simulink model "BEML_EMU"  (R2019b)
settings: configuration reference "ConfigSet_SimIntegration" (kept outside this file)
model workspace (MAT data in the model file):
  BrakesSampleTime = 0.01
  ConfigSampleTime = 0.05
  CouplingSampleTime = 0.05
  DoorsSampleTime = 0.05
  DynamicsSampleTime = 0.001
  ElectricalSampleTime = 0.05
  PRM_SimIntegration : Simulink.Parameter (value not decoded)
  PantographSampleTime = 0.05
  PneumaticsSampleTime = 0.01
  SampleTime = 0.001
  TractionSampleTime = 0.01
undefined symbols (not defined in the file): Acceleration, AngularAcceleration, AngularVelocity, BrakeFadeEnable, Brakes, BrakeShoeCoefficientCalculationMethod, BrakeShoeFrictionCoeff, BrakeTemperatureEnable, Common, DampingAdjustmentDesignMass, DavisCoeffA1, DavisCoeffA2, DavisCoeffB1, DavisCoeffB2, DavisCoefficients, DavisCoeffLeadCarC, DavisCoeffTailCarC, DiscIntNeverNeededParam, Doors, DragCalculationMethod, Dynamics, Effects, Electrical, EnableDampingAdjustmentByMass, Environment, Equipment, ExternalEffects, H, HasMotor, HasPanto, HornActivation, IsFirstVehicle, IsLastVehicle, isLeft, IsNonCab, LateralJolt, Location, LongitudinalJolt, MaxVehicles, MotionBaseSafetyCutout, OrientationDCM, P, Pantograph, Pneumatics, PneumaticsPoweredPanto, R, Traction, Transform, Tuning, UnitConfig, Velocity, VerticalJolt, VerticalJoltDown, VigilanceIntervention
libraries: simulink x35, IOStateMachinesLib x26, TestBenchLib x6, LatchesLib x3, BEML_EMU_BrakesInput_Lib x1, BEML_EMU_CBTCInterface_Lib x1, BEML_EMU_Couplers_Lib x1, BEML_EMU_DoorsInput_Lib x1, BEML_EMU_DynamicsInput_Lib x1, BEML_EMU_ElectricalInput_Lib x1, BEML_EMU_PantographInput_Lib x1, BEML_EMU_PneumaticsInput_Lib x1
(part 4 of 6)

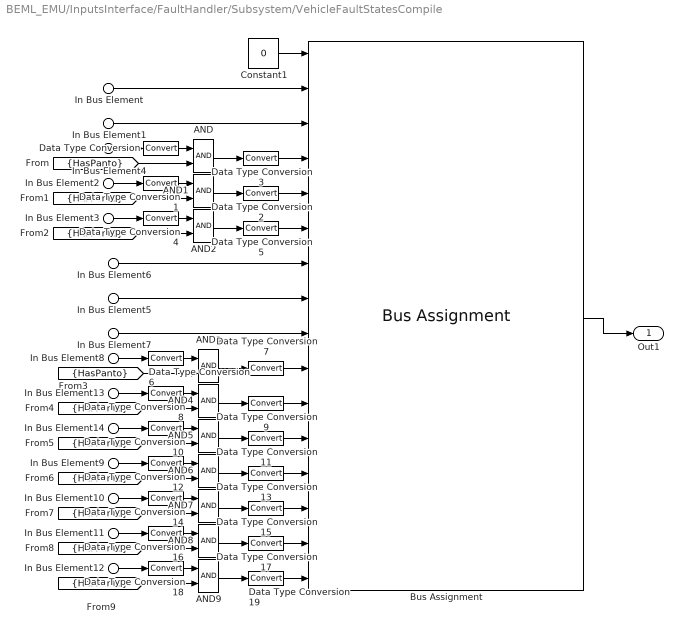
== system BEML_EMU/InputsInterface/FaultHandler/Subsystem/VehicleFaultStatesCompile ==
  In Bus Element : Inport  PortName=VehicleFaults  Element=DoorFaults.ObjectObstructingDoorWhileClosing
  In Bus Element1 : Inport  PortName=VehicleFaults  Element=DoorFaults.ObjectObstructingDoorWhileOpening
  In Bus Element4 : Inport  PortName=VehicleFaults  Element=ElectricalFaults.PantographDownForADDIntervention
  In Bus Element2 : Inport  PortName=VehicleFaults  Element=ElectricalFaults.PantographDownForORDIntervention
  In Bus Element3 : Inport  PortName=VehicleFaults  Element=ElectricalFaults.PantographRisingFailure
  In Bus Element6 : Inport  PortName=VehicleFaults  Element=ElectricalFaults.CCDetectedEmerDoorOpen
  In Bus Element7 : Inport  PortName=VehicleFaults  Element=ElectricalFaults.HVAC1EmergencyInverterTrip
  In Bus Element8 : Inport  PortName=VehicleFaults  Element=ElectricalFaults.VCBOpenedByACOvercurrent
  In Bus Element9 : Inport  PortName=VehicleFaults  Element=ElectricalFaults.VCBOpenedByMTrProtection
  In Bus Element10 : Inport  PortName=VehicleFaults  Element=ElectricalFaults.VCBOpenedByAPS
  In Bus Element11 : Inport  PortName=VehicleFaults  Element=ElectricalFaults.VCBMissingClosing
  In Bus Element12 : Inport  PortName=VehicleFaults  Element=ElectricalFaults.VCBMissingOpening
  In Bus Element13 : Inport  PortName=VehicleFaults  Element=ElectricalFaults.APSMCBGroupTripped
  In Bus Element14 : Inport  PortName=VehicleFaults  Element=ElectricalFaults.APSCircuitBreakerTripped
  In Bus Element5 : Inport  PortName=VehicleFaults  Element=TCMSFaults.MasterControllerandTrainLineIncongruence
  AND{,1..9} (10 alike) : Logic  AllPortsSameDT=off  OutDataTypeStr=boolean
  Bus Assignment : BusAssignment  AssignedSignals=DoorCloseObstruction,DoorOpenObstruction,PantographDownForADDIntervention,PantographDownForORDIntervention,PantographRaiseFailure,CCDetectDetrainmentDoorOpen,MasterControllerandTrainLineIncongruence,HVAC1EmergencyInverterTrip,VCBOpenedByACOvercurrent,MCBAPSGroupTripped,APSCircuitBreakerTripped,VCBOpenedByMTrProtection,VCBOpenedByAPS,VCBMissingClosing,VCBMissingOpening
  Constant1 : Constant  Value=0  OutDataTypeStr=Bus: BD_SimIntegration_Faults_Vehicle
  Data Type Conversion{,1..19} (20 alike) : DataTypeConversion
  Out1 : Outport
  wires:
  Constant1/1 -> Bus Assignment/1
  Bus Assignment/1 -> Out1/1
  In Bus Element/1 -> Bus Assignment/2
  In Bus Element1/1 -> Bus Assignment/3
  AND/1 -> Data Type Conversion3/1
  In Bus Element4/1 -> Data Type Conversion/1
  [HasPanto] -> AND/2
  [HasPanto] -> AND1/2
  AND1/1 -> Data Type Conversion2/1
  Data Type Conversion/1 -> AND/1
  Data Type Conversion1/1 -> AND1/1
  Data Type Conversion2/1 -> Bus Assignment/5
  Data Type Conversion3/1 -> Bus Assignment/4
  Data Type Conversion5/1 -> Bus Assignment/6
  Data Type Conversion4/1 -> AND2/1
  AND2/1 -> Data Type Conversion5/1
  In Bus Element3/1 -> Data Type Conversion4/1
  [HasPanto] -> AND2/2
  In Bus Element5/1 -> Bus Assignment/8
  In Bus Element6/1 -> Bus Assignment/7
  In Bus Element7/1 -> Bus Assignment/9
  [HasPanto] -> AND3/2
  In Bus Element8/1 -> Data Type Conversion6/1
  AND3/1 -> Data Type Conversion7/1
  Data Type Conversion6/1 -> AND3/1
  Data Type Conversion7/1 -> Bus Assignment/10
  Data Type Conversion9/1 -> Bus Assignment/11
  Data Type Conversion8/1 -> AND4/1
  AND4/1 -> Data Type Conversion9/1
  In Bus Element13/1 -> Data Type Conversion8/1
  [HasPanto] -> AND4/2
  [HasPanto] -> AND5/2
  In Bus Element14/1 -> Data Type Conversion10/1
  AND5/1 -> Data Type Conversion11/1
  Data Type Conversion10/1 -> AND5/1
  Data Type Conversion11/1 -> Bus Assignment/12
  Data Type Conversion13/1 -> Bus Assignment/13
  Data Type Conversion12/1 -> AND6/1
  AND6/1 -> Data Type Conversion13/1
  In Bus Element9/1 -> Data Type Conversion12/1
  [HasPanto] -> AND6/2
  [HasPanto] -> AND7/2
  In Bus Element10/1 -> Data Type Conversion14/1
  AND7/1 -> Data Type Conversion15/1
  Data Type Conversion14/1 -> AND7/1
  Data Type Conversion15/1 -> Bus Assignment/14
  Data Type Conversion17/1 -> Bus Assignment/15
  Data Type Conversion16/1 -> AND8/1
  AND8/1 -> Data Type Conversion17/1
  In Bus Element11/1 -> Data Type Conversion16/1
  [HasPanto] -> AND8/2
  [HasPanto] -> AND9/2
  In Bus Element12/1 -> Data Type Conversion18/1
  AND9/1 -> Data Type Conversion19/1
  Data Type Conversion18/1 -> AND9/1
  Data Type Conversion19/1 -> Bus Assignment/16
  In Bus Element2/1 -> Data Type Conversion1/1

== system BEML_EMU/InputsInterface/IOControlsInterface/InhibitsAndInternalRequests/Folding_Interlocks ==
  <RampWinder> : Inport
  RampSupport : Inport  Port=2
  GasSpring : Inport  Port=3
  <DummyCover> : Inport  Port=4
  Data Type Conversion1 : DataTypeConversion
  Data Type Conversion4 : DataTypeConversion
  NOT1 : Logic  Operator=NOT  AllPortsSameDT=off  OutDataTypeStr=boolean
  OR : Logic  Operator=OR  Inputs=3  AllPortsSameDT=off  OutDataTypeStr=boolean
  OR1 : Logic  Operator=OR  AllPortsSameDT=off  OutDataTypeStr=boolean
  InhibitDoorWinder : Outport
  InhibitRampWinder : Outport  Port=2
  wires:
  NOT1/1 -> OR1/1, OR/3
  Data Type Conversion4/1 -> InhibitDoorWinder/1
  OR/1 -> Data Type Conversion4/1
  <DummyCover>/1 -> NOT1/1
  Data Type Conversion1/1 -> InhibitRampWinder/1
  <RampWinder>/1 -> OR/2
  OR1/1 -> Data Type Conversion1/1
  RampSupport/1 -> OR1/2
  GasSpring/1 -> OR/1

== system BEML_EMU/InputsInterface/IOControlsInterface/InhibitsAndInternalRequests/Subsystem ==
  <ModeSelector> : Inport
  <ControlKey> : Inport  Port=2
  <MasterControllerHandle> : Inport  Port=3
  Compare To Constant1 : simulink/Logic and Bit Operations/Compare To Constant  relop===  const=1  OutDataTypeStr=boolean
  Compare To Constant2 : simulink/Logic and Bit Operations/Compare To Constant  relop===  const=-100  OutDataTypeStr=boolean
  Compare To Constant3 : simulink/Logic and Bit Operations/Compare To Constant  relop===  const=0  OutDataTypeStr=boolean
  Compare To Constant4 : simulink/Logic and Bit Operations/Compare To Constant  relop===  const=-100  OutDataTypeStr=boolean
  Compare To Constant5 : simulink/Logic and Bit Operations/Compare To Constant  relop===  const=0  OutDataTypeStr=boolean
  Compare To Constant6 : simulink/Logic and Bit Operations/Compare To Constant  relop===  const=5  OutDataTypeStr=boolean
  Data Type Conversion : DataTypeConversion
  Data Type Conversion1 : DataTypeConversion
  Data Type Conversion2 : DataTypeConversion
  Logical Operator1 : Logic  AllPortsSameDT=off  OutDataTypeStr=boolean
  Logical Operator2 : Logic  AllPortsSameDT=off  OutDataTypeStr=boolean
  Logical Operator3 : Logic  Operator=NOT  AllPortsSameDT=off  OutDataTypeStr=boolean
  Logical Operator4 : Logic  Operator=NOT  AllPortsSameDT=off  OutDataTypeStr=boolean
  Logical Operator5 : Logic  Operator=OR  AllPortsSameDT=off  OutDataTypeStr=boolean
  InhibitControlKey : Outport
  InhibitMS : Outport  Port=2
  InhibitMCH : Outport  Port=3
  wires:
  <ControlKey>/1 -> Compare To Constant1/1
  Compare To Constant6/1 -> Logical Operator5/2  "MS"
  Compare To Constant3/1 -> Logical Operator2/1  "MS"
  <ModeSelector>/1 -> Compare To Constant6/1, Compare To Constant5/1, Compare To Constant3/1
  Logical Operator1/1 -> Logical Operator4/1
  Logical Operator5/1 -> Data Type Conversion2/1
  Compare To Constant1/1 -> Logical Operator1/1  "Key"
  <MasterControllerHandle>/1 -> Compare To Constant4/1, Compare To Constant2/1
  Logical Operator4/1 -> Data Type Conversion1/1
  Compare To Constant2/1 -> Logical Operator1/2  "TBC"
  Logical Operator2/1 -> Logical Operator3/1
  Compare To Constant5/1 -> Logical Operator5/1  "MS"
  Logical Operator3/1 -> Data Type Conversion/1
  Compare To Constant4/1 -> Logical Operator2/2  "TBC"
  Data Type Conversion/1 -> InhibitControlKey/1
  Data Type Conversion1/1 -> InhibitMS/1
  Data Type Conversion2/1 -> InhibitMCH/1

== system BEML_EMU/InputsInterface/IOControlsInterface/InhibitsAndInternalRequests/Subsystem1 ==
  <Doors> : Inport  Partition=on  PartitionDimension=1  PartitionWidth=1  PartitionOffset=0
  Bus Selector3 : BusSelector  OutputSignals=OutputControlStates.DoorPosition
  Compare To Zero : simulink/Logic and Bit Operations/Compare To Zero  relop=>  OutDataTypeStr=boolean
  For Each : ForEach  DisableCoverage=on
  DoorsOpen : Outport  ConcatenationDimension=1
  wires:
  <Doors>/1 -> Bus Selector3/1
  Bus Selector3/1 -> Compare To Zero/1  "<DoorPosition>"
  Compare To Zero/1 -> DoorsOpen/1

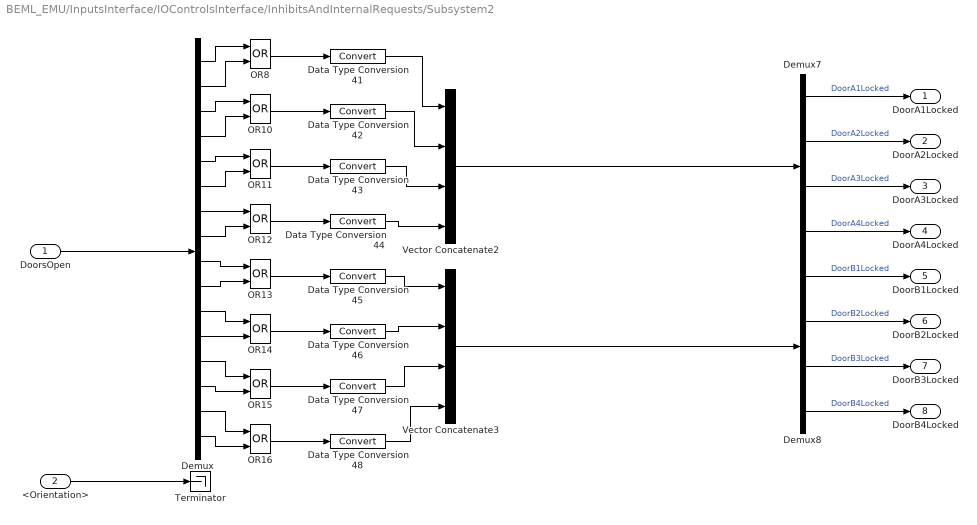
== system BEML_EMU/InputsInterface/IOControlsInterface/InhibitsAndInternalRequests/Subsystem2 ==
  DoorsOpen : Inport
  <Orientation> : Inport  Port=2
  Data Type Conversion{41..48} (8 alike) : DataTypeConversion
  Demux : Demux  Outputs=16
  Demux7 : Demux
  Demux8 : Demux
  OR{8,10..16} (8 alike) : Logic  Operator=OR  AllPortsSameDT=off  OutDataTypeStr=boolean
  Terminator : Terminator
  Vector Concatenate2 : Concatenate  NumInputs=4
  Vector Concatenate3 : Concatenate  NumInputs=4
  DoorA1Locked : Outport
  DoorA2Locked : Outport  Port=2
  DoorA3Locked : Outport  Port=3
  DoorA4Locked : Outport  Port=4
  DoorB1Locked : Outport  Port=5
  DoorB2Locked : Outport  Port=6
  DoorB3Locked : Outport  Port=7
  DoorB4Locked : Outport  Port=8
  wires:
  Demux/8 -> OR12/2
  OR13/1 -> Data Type Conversion45/1
  Data Type Conversion47/1 -> Vector Concatenate3/3
  Demux/2 -> OR8/2
  Demux/9 -> OR13/1
  Data Type Conversion48/1 -> Vector Concatenate3/4
  Demux/15 -> OR16/1
  Data Type Conversion46/1 -> Vector Concatenate3/2
  Demux/16 -> OR16/2
  Data Type Conversion45/1 -> Vector Concatenate3/1
  OR14/1 -> Data Type Conversion46/1
  Demux7/3 -> DoorA3Locked/1  "DoorA3Locked"
  Demux/4 -> OR10/2
  OR16/1 -> Data Type Conversion48/1
  Demux/10 -> OR13/2
  OR11/1 -> Data Type Conversion43/1
  Demux/11 -> OR14/1
  Demux8/1 -> DoorB1Locked/1  "DoorB1Locked"
  Demux7/4 -> DoorA4Locked/1  "DoorA4Locked"
  Demux/14 -> OR15/2
  Demux/7 -> OR12/1
  Demux/12 -> OR14/2
  Demux7/2 -> DoorA2Locked/1  "DoorA2Locked"
  Demux/6 -> OR11/2
  Demux/3 -> OR10/1
  Data Type Conversion41/1 -> Vector Concatenate2/1
  Demux/1 -> OR8/1
  Vector Concatenate2/1 -> Demux7/1
  Demux/5 -> OR11/1
  OR10/1 -> Data Type Conversion42/1
  OR8/1 -> Data Type Conversion41/1
  Demux8/4 -> DoorB4Locked/1  "DoorB4Locked"
  OR15/1 -> Data Type Conversion47/1
  Data Type Conversion42/1 -> Vector Concatenate2/2
  OR12/1 -> Data Type Conversion44/1
  Demux/13 -> OR15/1
  Vector Concatenate3/1 -> Demux8/1
  Demux8/3 -> DoorB3Locked/1  "DoorB3Locked"
  Data Type Conversion44/1 -> Vector Concatenate2/4
  Data Type Conversion43/1 -> Vector Concatenate2/3
  Demux8/2 -> DoorB2Locked/1  "DoorB2Locked"
  DoorsOpen/1 -> Demux/1
  <Orientation>/1 -> Terminator/1
  Demux7/1 -> DoorA1Locked/1  "DoorA1Locked"

== system BEML_EMU/InputsInterface/IOControlsInterface/InhibitsAndInternalRequests/Unfolding_interlocks ==
  note: when either of Winder is active, inhibit all the controls
  <RampCoverLockingLever> : Inport
  <SafetyCover> : Inport  Port=2
  <RampCover> : Inport  Port=3
  <DummyCover> : Inport  Port=4
  EDELR : Inport  Port=5
  AND : Logic  AllPortsSameDT=off  OutDataTypeStr=boolean
  Bus Selector : BusSelector  OutputSignals=Doors.EmerDoorLatched
  Data Type Conversion{,1..3} (4 alike) : DataTypeConversion
  NOT{,1..4} (5 alike) : Logic  Operator=NOT  AllPortsSameDT=off  OutDataTypeStr=boolean
  OR1 : Logic  Operator=OR  AllPortsSameDT=off  OutDataTypeStr=boolean
  InhibitSafetyCover : Outport  OutputWhenDisabled=reset  InitialOutput=1
  InhibitLockingLever : Outport  Port=2  OutputWhenDisabled=reset  InitialOutput=1
  InhibitRampCover : Outport  Port=3  OutputWhenDisabled=reset  InitialOutput=1
  InhibitRampHandle : Outport  Port=4  OutputWhenDisabled=reset  InitialOutput=1
  wires:
  <RampCover>/1 -> NOT2/1
  AND/1 -> NOT1/1
  <SafetyCover>/1 -> OR1/2, AND/1
  EDELR/1 -> Bus Selector/1
  <DummyCover>/1 -> NOT/1
  <RampCoverLockingLever>/1 -> NOT3/1
  NOT/1 -> OR1/1
  OR1/1 -> Data Type Conversion/1
  NOT2/1 -> Data Type Conversion2/1
  NOT3/1 -> Data Type Conversion3/1
  NOT1/1 -> Data Type Conversion1/1
  Data Type Conversion/1 -> InhibitSafetyCover/1
  Data Type Conversion2/1 -> InhibitRampHandle/1
  Data Type Conversion3/1 -> InhibitRampCover/1
  Data Type Conversion1/1 -> InhibitLockingLever/1
  NOT4/1 -> AND/2
  Bus Selector/1 -> NOT4/1  "<EmerDoorLatched>"

== system BEML_EMU/InputsInterface/VehicleConfigProcessing/VehicleConfigInterface/VehicleConfigInterface ==
  VehicleConfig : Inport  Partition=on  PartitionDimension=1  PartitionWidth=1  PartitionOffset=0
  VehicleUpEnabled : Inport  Port=2  Partition=on  PartitionDimension=1  PartitionWidth=1  PartitionOffset=0
  VehicleDownEnabled : Inport  Port=3  Partition=on  PartitionDimension=1  PartitionWidth=1  PartitionOffset=0
  ClassDown : Inport  Port=4  Partition=on  PartitionDimension=1  PartitionWidth=1  PartitionOffset=0
  ClassUp : Inport  Port=5  Partition=on  PartitionDimension=1  PartitionWidth=1  PartitionOffset=0
  TrainInput : Inport  Port=6
  UnitID : Inport  Port=7  Partition=on  PartitionDimension=1  PartitionWidth=1  PartitionOffset=0
  MaxUnits : Inport  Port=8
  AssignBrakes : Subsystem
  AssignDoors : Subsystem
  AssignElectrical : Subsystem
  AssignEquipment : Subsystem
  AssignPanto : Subsystem
  AssignPneumatics : Subsystem
  AssignTraction : Subsystem
  Bus Assignment1 : BusAssignment  AssignedSignals=Common,Location,Dynamics,Brakes,Pneumatics,Traction,Pantograph,Doors,Electrical,Equipment
  Bus Selector : BusSelector  OutputSignals=Dynamics
  Bus Selector1 : BusSelector  OutputSignals=Common
  Bus Selector2 : BusSelector  OutputSignals=Common.Enabled
  Bus Selector4 : BusSelector  OutputSignals=Brakes
  Common : Subsystem
  Constant1 : Constant  Value=0  OutDataTypeStr=Bus: BD_SimIntegration_Cfg_Vehicle
  Dynamics : Subsystem
  For Each : ForEach  DisableCoverage=on  ShowIterationIndex=on
  LocationConfig : Subsystem
  VehicleConfigProcessed : Outport  ConcatenationDimension=1  VectorParamsAs1DForOutWhenUnconnected=off
  Enable : Outport  Port=2  ConcatenationDimension=1
  UnitConn : Outport  Port=3  ConcatenationDimension=1
  wires:
  Bus Selector4/1 -> AssignBrakes/1(Input)  "<Brakes>"
  Bus Selector1/1 -> Common/1(Input)  "<Common>"
  TrainInput/1 -> Dynamics/2(TrainInput)
  Dynamics/1(DynamicsProcessed) -> Bus Assignment1/4  "Dynamics"
  LocationConfig/1(LocationConfig) -> Bus Assignment1/3  "Location"
  VehicleDownEnabled/1 -> LocationConfig/3(VehicleEnabledDown)
  VehicleUpEnabled/1 -> LocationConfig/2(VehicleEnabledUp)
  Bus Selector2/1 -> LocationConfig/1(VehicleEnabled)  "<Enabled>"
  Bus Selector/1 -> Dynamics/1(Dynamics)  "<Dynamics>"
  Constant1/1 -> Bus Assignment1/1
  Bus Assignment1/1 -> VehicleConfigProcessed/1  "VehicleConfig"
  VehicleConfig/1 -> AssignPneumatics/1(VehicleConfig), AssignTraction/1(VehicleConfig), AssignPanto/1(VehicleConfig), AssignDoors/1(VehicleConfig), AssignEquipment/1(VehicleConfig), AssignElectrical/1(VehicleConfig), Bus Selector4/1, Bus Selector/1, LocationConfig/7(VehicleConfig), Bus Selector2/1, Bus Selector1/1
  AssignBrakes/1(EquipmentBus) -> Bus Assignment1/5  "Brakes"
  AssignPneumatics/1(PneumaticsBus) -> Bus Assignment1/6  "Pneumatics"
  AssignTraction/1(TractionBus) -> Bus Assignment1/7  "Traction"
  AssignPanto/1(PantoBus) -> Bus Assignment1/8  "Pantograph"
  AssignElectrical/1(ElectricalBus) -> Bus Assignment1/10  "Electrical"
  AssignDoors/1(Doors) -> Bus Assignment1/9
  AssignEquipment/1(EquipmentBus) -> Bus Assignment1/11  "Equipment"
  For Each/1 -> AssignElectrical/2(Index)
  ClassDown/1 -> LocationConfig/4(ClassDown)
  ClassUp/1 -> LocationConfig/5(ClassUp)
  LocationConfig/2(Enabled) -> Enable/1
  LocationConfig/3(UnitConnection) -> UnitConn/1
  UnitID/1 -> LocationConfig/6(UnitID)
  Common/1(Common) -> Bus Assignment1/2  "Brakes"
  MaxUnits/1 -> LocationConfig/8(MaxUnit)

== system BEML_EMU/InputsInterface/VehicleConfigProcessing/VehicleConfigInterface/VehicleEnabled ==
  VehicleConfig : Inport
  Constant : Constant  Value=false  OutDataTypeStr=boolean
  Constant1 : Constant  Value=0  OutDataTypeStr=int32
  Data Type Conversion : DataTypeConversion  OutDataTypeStr=int32
  SelectDown : Selector  InputPortWidth=MaxVehicles+2  IndexOptions=Starting index (dialog)  Indices=3  OutputSizes=MaxVehicles
  SelectDown1 : Selector  InputPortWidth=MaxVehicles+2  IndexOptions=Starting index (dialog)  Indices=3  OutputSizes=MaxVehicles
  SelectUp : Selector  InputPortWidth=MaxVehicles+2  IndexOptions=Starting index (dialog)  Indices=1  OutputSizes=MaxVehicles
  SelectUp1 : Selector  InputPortWidth=MaxVehicles+2  IndexOptions=Starting index (dialog)  Indices=1  OutputSizes=MaxVehicles
  Subsystem : Subsystem
  Subsystem1 : Subsystem
  Vector Concatenate : Concatenate  NumInputs=3
  Vector Concatenate1 : Concatenate  NumInputs=3
  VehicleEnabledUp : Outport  VectorParamsAs1DForOutWhenUnconnected=off
  VehicleEnabledDown : Outport  Port=2  VectorParamsAs1DForOutWhenUnconnected=off
  VehicleClassDown : Outport  Port=3  VectorParamsAs1DForOutWhenUnconnected=off
  VehicleClassUp : Outport  Port=4  VectorParamsAs1DForOutWhenUnconnected=off
  wires:
  SelectUp/1 -> VehicleEnabledUp/1
  SelectDown/1 -> VehicleEnabledDown/1
  Subsystem/1(Enabled) -> Vector Concatenate/2
  Vector Concatenate/1 -> SelectDown/1, SelectUp/1
  Constant/1 -> Vector Concatenate/3, Vector Concatenate/1
  VehicleConfig/1 -> Subsystem1/1(VehicleConfig), Subsystem/1(VehicleConfig)
  Subsystem1/1(Class) -> Data Type Conversion/1
  Vector Concatenate1/1 -> SelectDown1/1, SelectUp1/1
  SelectDown1/1 -> VehicleClassDown/1
  Data Type Conversion/1 -> Vector Concatenate1/2
  Constant1/1 -> Vector Concatenate1/3, Vector Concatenate1/1
  SelectUp1/1 -> VehicleClassUp/1

== system BEML_EMU/SimulatorSystems/AudioSystemInterface/Subsystem1/For Each Subsystem ==
  Doors : Inport  Partition=on  PartitionDimension=1  PartitionWidth=1  PartitionOffset=0
  Bus Selector : BusSelector  OutputSignals=Audio.DoorOpening,Audio.DoorClosing,Audio.DoorOpeningAlarm,Audio.DoorClosingAlarm,Audio.DoorEmergencyReleased
  For Each : ForEach  DisableCoverage=on
  OR : Logic  Operator=OR  AllPortsSameDT=off  OutDataTypeStr=boolean
  Opening : Outport  ConcatenationDimension=1
  Closing : Outport  Port=2  ConcatenationDimension=1
  OpeningorClosingAlarm : Outport  Port=3  ConcatenationDimension=1
  EED_EADOperated : Outport  Port=4  ConcatenationDimension=1
  wires:
  Doors/1 -> Bus Selector/1
  Bus Selector/1 -> Opening/1  "<DoorOpening>"
  Bus Selector/2 -> Closing/1  "<DoorClosing>"
  OR/1 -> OpeningorClosingAlarm/1
  Bus Selector/3 -> OR/1  "<DoorOpeningAlarm>"
  Bus Selector/4 -> OR/2  "<DoorClosingAlarm>"
  Bus Selector/5 -> EED_EADOperated/1  "<DoorEmergencyReleased>"

== system BEML_EMU/SimulatorSystems/AudioSystemInterface/Subsystem1/For Each Subsystem1 ==
  Traction : Inport  Partition=on  PartitionDimension=1  PartitionWidth=1  PartitionOffset=0
  Bus Selector1 : BusSelector  OutputSignals=TCUSlipDetected,TCUSlideDetected
  For Each : ForEach  DisableCoverage=on
  Slip : Outport  ConcatenationDimension=1
  Slide : Outport  Port=2  ConcatenationDimension=1
  wires:
  Bus Selector1/2 -> Slide/1  "<TCUSlideDetected>"
  Traction/1 -> Bus Selector1/1
  Bus Selector1/1 -> Slip/1  "<TCUSlipDetected>"

== system BEML_EMU/SimulatorSystems/AudioSystemInterface/Subsystem1/For Each Subsystem2 ==
  Axle : Inport  Partition=on  PartitionDimension=1  PartitionWidth=1  PartitionOffset=0
  Bus Selector : BusSelector  OutputSignals=BrakeCylinderPressures
  For Each : ForEach  DisableCoverage=on
  BCPressures : Outport  ConcatenationDimension=1
  wires:
  Bus Selector/1 -> BCPressures/1  "<BrakeCylinderPressures>"
  Axle/1 -> Bus Selector/1

== system BEML_EMU/SimulatorSystems/AudioSystemInterface/Subsystem1/Subsystem1 ==
  <Inertia> : Inport
  Slip : Inport  Port=2
  Slide : Inport  Port=3
  Abs1 : Abs
  Bus Selector6 : BusSelector  OutputSignals=Velocity
  Compare To Constant1 : simulink/Logic and Bit Operations/Compare To Constant  relop=>  const=1.4  OutDataTypeStr=boolean
  Data Type Conversion18 : DataTypeConversion  OutDataTypeStr=double
  Data Type Conversion19 : DataTypeConversion  OutDataTypeStr=double
  Detect Increase : simulink/Logic and Bit Operations/Detect Increase  vinit=0.0  OutDataTypeStr=boolean
  Logical Operator2 : Logic  AllPortsSameDT=off  OutDataTypeStr=boolean
  Logical Operator3 : Logic  Inputs=3  AllPortsSameDT=off  OutDataTypeStr=boolean
  SlipSound : Outport
  SlideSound : Outport  Port=2
  wires:
  Logical Operator3/1 -> Data Type Conversion18/1
  Abs1/1 -> Detect Increase/1, Compare To Constant1/1
  Compare To Constant1/1 -> Logical Operator3/3, Logical Operator2/1
  Detect Increase/1 -> Logical Operator3/2
  Bus Selector6/1 -> Abs1/1  "<Velocity>"
  Logical Operator2/1 -> Data Type Conversion19/1
  Slip/1 -> Logical Operator3/1
  Data Type Conversion18/1 -> SlipSound/1
  <Inertia>/1 -> Bus Selector6/1
  Data Type Conversion19/1 -> SlideSound/1
  Slide/1 -> Logical Operator2/2

== system BEML_EMU/SimulatorSystems/ScoringSystemInterface/TrainLevelScoring/For Each Subsystem ==
  In1 : Inport  Partition=on  PartitionDimension=1  PartitionWidth=1  PartitionOffset=0
  Bus Selector : BusSelector  OutputSignals=TractionControl.TCMS
  For Each : ForEach  DisableCoverage=on
  Subsystem : Subsystem
  Sum of Elements : Sum  Inputs=+
  Sum of Elements1 : Sum  Inputs=+
  VehicleTractiveEnergy : Outport  ConcatenationDimension=1
  VehicleEDBrakingEnergy : Outport  Port=2  ConcatenationDimension=1
  wires:
  In1/1 -> Bus Selector/1
  Bus Selector/1 -> Subsystem/1(<Bogie>)  "<TCMS>"
  Subsystem/1(Out1) -> Sum of Elements/1
  Sum of Elements/1 -> VehicleTractiveEnergy/1
  Sum of Elements1/1 -> VehicleEDBrakingEnergy/1
  Subsystem/2(Out2) -> Sum of Elements1/1

== system BEML_EMU/SimulatorSystems/ScoringSystemInterface/TrainLevelScoring/For Each Subsystem1 ==
  In1 : Inport  Partition=on  PartitionDimension=1  PartitionWidth=1  PartitionOffset=0
  Bus Selector : BusSelector  OutputSignals=OutputControlStates.AuxModuleON
  For Each : ForEach  DisableCoverage=on
  Out1 : Outport  ConcatenationDimension=1
  wires:
  In1/1 -> Bus Selector/1
  Bus Selector/1 -> Out1/1  "<AuxModuleON>"

== system BEML_EMU/SimulatorSystems/Subsystem/Input Adapter/MotionBaseInputAdapter ==
  VehicleInput : Inport
  DynamicsInput : Inport  Port=2
  MotionBaseInputs : Inport  Port=3
  BinarySwitch : TestBenchLib/BinarySwitch  value=1  init_value=1  block_colour=[0 1 0]  WorkspaceVarName=0
      settings: SourceProductName=Sydac Utilities
  Bus Assignment : BusAssignment  AssignedSignals=Dynamics,Effects,Environment,Tuning,MotionBaseSafetyCutout
  Constant6 : Constant  Value=0  OutDataTypeStr=Bus: BD_MotionBase_In_Vehicle
  Data Type Conversion : DataTypeConversion
  Effects In Processing : Subsystem
  Environment Dynamics In Processing : Subsystem
  Tuning In Processing : Subsystem
  Vehicle Dynamics In Processing : Subsystem
  MotionBaseInput : Outport
  wires:
  Constant6/1 -> Bus Assignment/1
  Bus Assignment/1 -> MotionBaseInput/1
  Vehicle Dynamics In Processing/1(VehicleDynamics) -> Bus Assignment/2
  VehicleInput/1 -> Vehicle Dynamics In Processing/1(VehicleInput)
  DynamicsInput/1 -> Vehicle Dynamics In Processing/2(DynamicsInput)
  Environment Dynamics In Processing/1(Environment) -> Bus Assignment/4
  Effects In Processing/1(Effects) -> Bus Assignment/3
  BinarySwitch/1 -> Data Type Conversion/1
  Tuning In Processing/1(Environment) -> Bus Assignment/5
  Data Type Conversion/1 -> Bus Assignment/6
  MotionBaseInputs/1 -> Effects In Processing/1(MotionBaseInput), Tuning In Processing/1(MotionBaseInput)

== system BEML_EMU/InputsInterface/FaultHandler/Subsystem/Subsystem/Subsystem ==
  In Bus Element28 : Inport  PortName=InputControlStates  Element=OCCB1
  In Bus Element29 : Inport  PortName=InputControlStates  Element=OCCB2
  In Bus Element30 : Inport  PortName=InputControlStates  Element=PISCB1
  In Bus Element31 : Inport  PortName=InputControlStates  Element=PISCB2
  AND : Logic  Inputs=4  AllPortsSameDT=off  OutDataTypeStr=boolean
  Out1 : Outport
  wires:
  AND/1 -> Out1/1
  In Bus Element29/1 -> AND/2
  In Bus Element30/1 -> AND/3
  In Bus Element28/1 -> AND/1
  In Bus Element31/1 -> AND/4

== system BEML_EMU/InputsInterface/FaultHandler/Subsystem/Subsystem/Subsystem1 ==
  In Bus Element : Inport  PortName=InputControlStates  Element=TBCCB1
  In Bus Element1 : Inport  PortName=InputControlStates  Element=TBCCB2
  In Bus Element2 : Inport  PortName=InputControlStates  Element=SSICB
  In Bus Element3 : Inport  PortName=InputControlStates  Element=HCB
  In Bus Element4 : Inport  PortName=InputControlStates  Element=POCB
  In Bus Element5 : Inport  PortName=InputControlStates  Element=TVDUCB
  In Bus Element6 : Inport  PortName=InputControlStates  Element=ODDCB
  In Bus Element7 : Inport  PortName=InputControlStates  Element=WIFICB
  In Bus Element8 : Inport  PortName=InputControlStates  Element=WFLCB
  In Bus Element9 : Inport  PortName=InputControlStates  Element=WWCB
  In Bus Element10 : Inport  PortName=InputControlStates  Element=VCBCB
  AND : Logic  Inputs=11  AllPortsSameDT=off  OutDataTypeStr=boolean
  Out1 : Outport
  wires:
  AND/1 -> Out1/1
  In Bus Element1/1 -> AND/2
  In Bus Element/1 -> AND/1
  In Bus Element2/1 -> AND/3
  In Bus Element3/1 -> AND/4
  In Bus Element4/1 -> AND/5
  In Bus Element5/1 -> AND/6
  In Bus Element6/1 -> AND/7
  In Bus Element7/1 -> AND/8
  In Bus Element8/1 -> AND/9
  In Bus Element9/1 -> AND/10
  In Bus Element10/1 -> AND/11

== system BEML_EMU/InputsInterface/FaultHandler/Subsystem/Subsystem/Subsystem2 ==
  In Bus Element : Inport  PortName=InputControlStates  Element=MLCB
  In Bus Element1 : Inport  PortName=InputControlStates  Element=CELCB
  In Bus Element2 : Inport  PortName=InputControlStates  Element=HLLCB
  In Bus Element3 : Inport  PortName=InputControlStates  Element=HLRCB
  In Bus Element4 : Inport  PortName=InputControlStates  Element=TLLCB
  In Bus Element5 : Inport  PortName=InputControlStates  Element=TLRCB
  In Bus Element6 : Inport  PortName=InputControlStates  Element=CILCB
  AND : Logic  Inputs=7  AllPortsSameDT=off  OutDataTypeStr=boolean
  Out1 : Outport
  wires:
  AND/1 -> Out1/1
  In Bus Element/1 -> AND/1
  In Bus Element1/1 -> AND/2
  In Bus Element2/1 -> AND/3
  In Bus Element3/1 -> AND/4
  In Bus Element4/1 -> AND/5
  In Bus Element5/1 -> AND/6
  In Bus Element6/1 -> AND/7

== system BEML_EMU/InputsInterface/FaultHandler/Subsystem/Subsystem/Subsystem3 ==
  In Bus Element : Inport  PortName=InputControlStates  Element=ELCB1
  In Bus Element1 : Inport  PortName=InputControlStates  Element=ELCB2
  In Bus Element2 : Inport  PortName=InputControlStates  Element=ILCB1
  In Bus Element3 : Inport  PortName=InputControlStates  Element=ILCB2
  AND : Logic  Inputs=4  AllPortsSameDT=off  OutDataTypeStr=boolean
  Out1 : Outport
  wires:
  AND/1 -> Out1/1
  In Bus Element/1 -> AND/1
  In Bus Element1/1 -> AND/2
  In Bus Element2/1 -> AND/3
  In Bus Element3/1 -> AND/4

== system BEML_EMU/InputsInterface/FaultHandler/Subsystem/Subsystem/Subsystem4 ==
  In Bus Element : Inport  PortName=InputControlStates  Element=LDICB
  In Bus Element1 : Inport  PortName=InputControlStates  Element=LDLCB
  In Bus Element2 : Inport  PortName=InputControlStates  Element=LDRCB
  In Bus Element3 : Inport  PortName=InputControlStates  Element=DLCB
  In Bus Element4 : Inport  PortName=InputControlStates  Element=DRCB
  In Bus Element5 : Inport  PortName=InputControlStates  Element=DPLCB
  In Bus Element6 : Inport  PortName=InputControlStates  Element=EDCB
  AND : Logic  Inputs=7  AllPortsSameDT=off  OutDataTypeStr=boolean
  Out1 : Outport
  wires:
  AND/1 -> Out1/1
  In Bus Element2/1 -> AND/1
  In Bus Element1/1 -> AND/2
  In Bus Element3/1 -> AND/3
  In Bus Element4/1 -> AND/4
  In Bus Element/1 -> AND/5
  In Bus Element5/1 -> AND/6
  In Bus Element6/1 -> AND/7

== system BEML_EMU/InputsInterface/FaultHandler/Subsystem/Subsystem/Subsystem5 ==
  In Bus Element : Inport  PortName=InputControlStates  Element=BLCB
  In Bus Element1 : Inport  PortName=InputControlStates  Element=CMCCB
  In Bus Element2 : Inport  PortName=InputControlStates  Element=ZVBACB
  In Bus Element3 : Inport  PortName=InputControlStates  Element=EBLR2CB
  In Bus Element4 : Inport  PortName=InputControlStates  Element=EBLR1CB
  In Bus Element5 : Inport  PortName=InputControlStates  Element=EBMVCB
  In Bus Element6 : Inport  PortName=InputControlStates  Element=PBCB
  In Bus Element7 : Inport  PortName=InputControlStates  Element=BECUCB1
  In Bus Element8 : Inport  PortName=InputControlStates  Element=BECUCB2
  In Bus Element9 : Inport  PortName=InputControlStates  Element=BECUCB3
  AND : Logic  Inputs=10  AllPortsSameDT=off  OutDataTypeStr=boolean
  Out1 : Outport
  wires:
  AND/1 -> Out1/1
  In Bus Element/1 -> AND/1
  In Bus Element1/1 -> AND/2
  In Bus Element2/1 -> AND/3
  In Bus Element4/1 -> AND/4
  In Bus Element3/1 -> AND/5
  In Bus Element5/1 -> AND/6
  In Bus Element6/1 -> AND/7
  In Bus Element7/1 -> AND/8
  In Bus Element8/1 -> AND/9
  In Bus Element9/1 -> AND/10

== system BEML_EMU/InputsInterface/FaultHandler/Subsystem/Subsystem/Subsystem6 ==
  In Bus Element : Inport  PortName=InputControlStates  Element=BCGCB
  In Bus Element1 : Inport  PortName=InputControlStates  Element=APSCB
  AND : Logic  AllPortsSameDT=off  OutDataTypeStr=boolean
  Out1 : Outport
  wires:
  AND/1 -> Out1/1
  In Bus Element/1 -> AND/1
  In Bus Element1/1 -> AND/2

== system BEML_EMU/InputsInterface/FaultHandler/Subsystem/Subsystem/Subsystem7 ==
  In Bus Element : Inport  PortName=InputControlStates  Element=TDICB
  In Bus Element1 : Inport  PortName=InputControlStates  Element=CDUCB
  In Bus Element2 : Inport  PortName=InputControlStates  Element=ERCB
  In Bus Element3 : Inport  PortName=InputControlStates  Element=RIO1CB
  In Bus Element4 : Inport  PortName=InputControlStates  Element=RIO2CB
  In Bus Element5 : Inport  PortName=InputControlStates  Element=SIOCB1
  In Bus Element6 : Inport  PortName=InputControlStates  Element=SIOCB2
  In Bus Element7 : Inport  PortName=InputControlStates  Element=DIOCB2
  In Bus Element8 : Inport  PortName=InputControlStates  Element=DIOCB1
  In Bus Element9 : Inport  PortName=InputControlStates  Element=CSCCB
  In Bus Element10 : Inport  PortName=InputControlStates  Element=CSBCB
  In Bus Element11 : Inport  PortName=InputControlStates  Element=CSACB
  In Bus Element12 : Inport  PortName=InputControlStates  Element=TBNCB
  AND : Logic  Inputs=15  AllPortsSameDT=off  OutDataTypeStr=boolean
  CDUCB1_FixMe : Constant
  ERCB1_FixMe1 : Constant
  Out1 : Outport
  wires:
  In Bus Element/1 -> AND/1
  AND/1 -> Out1/1
  CDUCB1_FixMe/1 -> AND/2
  ERCB1_FixMe1/1 -> AND/3
  In Bus Element3/1 -> AND/4
  In Bus Element4/1 -> AND/5
  In Bus Element5/1 -> AND/6
  In Bus Element6/1 -> AND/7
  In Bus Element8/1 -> AND/8
  In Bus Element7/1 -> AND/9
  In Bus Element1/1 -> AND/10
  In Bus Element9/1 -> AND/11
  In Bus Element10/1 -> AND/12
  In Bus Element11/1 -> AND/13
  In Bus Element12/1 -> AND/14
  In Bus Element2/1 -> AND/15

== system BEML_EMU/InputsInterface/FaultHandler/Subsystem/Subsystem/Subsystem8 ==
  In Bus Element : Inport  PortName=InputControlStates  Element=TRIVCB
  In Bus Element1 : Inport  PortName=InputControlStates  Element=VIO2CB
  In Bus Element2 : Inport  PortName=InputControlStates  Element=VIO1CB
  In Bus Element3 : Inport  PortName=InputControlStates  Element=PPU1CB
  In Bus Element4 : Inport  PortName=InputControlStates  Element=PPU2CB
  In Bus Element5 : Inport  PortName=InputControlStates  Element=PPU3CB
  In Bus Element6 : Inport  PortName=InputControlStates  Element=C1CB
  In Bus Element7 : Inport  PortName=InputControlStates  Element=NBCB
  In Bus Element8 : Inport  PortName=InputControlStates  Element=MMCB
  In Bus Element9 : Inport  PortName=InputControlStates  Element=CRSBCB
  In Bus Element10 : Inport  PortName=InputControlStates  Element=DMICB
  In Bus Element11 : Inport  PortName=InputControlStates  Element=CBTCCB1
  In Bus Element12 : Inport  PortName=InputControlStates  Element=NVICB
  In Bus Element13 : Inport  PortName=InputControlStates  Element=CCNVIO1CB
  In Bus Element14 : Inport  PortName=InputControlStates  Element=TWVCB
  AND : Logic  Inputs=16  AllPortsSameDT=off  OutDataTypeStr=boolean
  CRSACB_FixME : Constant
  Out1 : Outport
  wires:
  AND/1 -> Out1/1
  In Bus Element/1 -> AND/1
  In Bus Element1/1 -> AND/2
  In Bus Element2/1 -> AND/3
  In Bus Element5/1 -> AND/4
  In Bus Element4/1 -> AND/5
  In Bus Element3/1 -> AND/6
  In Bus Element6/1 -> AND/7
  In Bus Element7/1 -> AND/8
  In Bus Element8/1 -> AND/9
  In Bus Element9/1 -> AND/10
  In Bus Element10/1 -> AND/12
  In Bus Element11/1 -> AND/14
  In Bus Element12/1 -> AND/15
  In Bus Element13/1 -> AND/16
  CRSACB_FixME/1 -> AND/11
  In Bus Element14/1 -> AND/13

== system BEML_EMU/InputsInterface/FaultHandler/Subsystem/Subsystem/Subsystem9 ==
  In Bus Element15 : Inport  PortName=InputControlStates  Element=CBFCCB
  In Bus Element16 : Inport  PortName=InputControlStates  Element=SAC2CCB
  In Bus Element17 : Inport  PortName=InputControlStates  Element=SAC1CCB
  AND : Logic  Inputs=3  AllPortsSameDT=off  OutDataTypeStr=boolean
  Out1 : Outport
  wires:
  AND/1 -> Out1/1
  In Bus Element15/1 -> AND/1
  In Bus Element16/1 -> AND/2
  In Bus Element17/1 -> AND/3

== system BEML_EMU/InputsInterface/VehicleConfigProcessing/VehicleConfigInterface/VehicleConfigInterface/AssignBrakes ==
  Input : Inport
  Bus Assignment3 : BusAssignment  AssignedSignals=BrakeShoeFrictionCoeff,BrakeShoeCoefficientCalculationMethod,BrakeFadeEnable,BrakeTemperatureEnable
  Bus Selector : BusSelector  OutputSignals=BrakeShoeCoefficientCalculationMethod,BrakeFadeEnable,BrakeTemperatureEnable
  Constant1 : Constant  Value=0.29  OutDataTypeStr=Inherit: Inherit via back propagation
  Constant6 : Constant  Value=0  OutDataTypeStr=Bus: BD_TrainBrakes_Cfg_Vehicle
  Data Type Conversion3 : DataTypeConversion
  EquipmentBus : Outport  VectorParamsAs1DForOutWhenUnconnected=off
  wires:
  Bus Assignment3/1 -> EquipmentBus/1
  Constant6/1 -> Bus Assignment3/1
  Data Type Conversion3/1 -> Bus Assignment3/2
  Constant1/1 -> Data Type Conversion3/1
  Input/1 -> Bus Selector/1
  Bus Selector/1 -> Bus Assignment3/3  "<BrakeShoeCoefficientCalculationMethod>"
  Bus Selector/2 -> Bus Assignment3/4  "<BrakeFadeEnable>"
  Bus Selector/3 -> Bus Assignment3/5  "<BrakeTemperatureEnable>"

== system BEML_EMU/InputsInterface/VehicleConfigProcessing/VehicleConfigInterface/VehicleConfigInterface/AssignDoors ==
  In Bus Element : Inport  PortName=VehicleConfig  Element=Common.Class
  Data Type Conversion : DataTypeConversion
  Merge1 : Merge  Inputs=4
  Switch Case2 : SwitchCase  CaseConditions={[101], [102], [103]}
  VehicleEquipment1 : Subsystem  mask(Tram Vehicle Equipment){IsLeft=off, NumberOfDoors=8}
      mask prompts: IsLeft "IsLeft Door?"; NumberOfDoors "Number Of Doors"
      mask DialogControl ParameterGroupVar Prompt: Equipment
  VehicleEquipment2 : Subsystem  mask(Tram Vehicle Equipment){IsLeft=off, NumberOfDoors=8}
      mask prompts: IsLeft "IsLeft Door?"; NumberOfDoors "Number Of Doors"
      mask DialogControl ParameterGroupVar Prompt: Equipment
  VehicleEquipment3 : Subsystem  mask(Tram Vehicle Equipment){IsLeft=off, NumberOfDoors=0}
      mask prompts: IsLeft "IsLeft Door?"; NumberOfDoors "Number Of Doors"
      mask DialogControl ParameterGroupVar Prompt: Equipment
  VehicleEquipment4 : Subsystem  mask(Tram Vehicle Equipment){IsLeft=off, NumberOfDoors=8}
      mask prompts: IsLeft "IsLeft Door?"; NumberOfDoors "Number Of Doors"
      mask DialogControl ParameterGroupVar Prompt: Equipment
  Doors : Outport  VectorParamsAs1DForOutWhenUnconnected=off
  wires:
  VehicleEquipment2/1(EquipmentBus) -> Merge1/3
  VehicleEquipment1/1(EquipmentBus) -> Merge1/2
  VehicleEquipment3/1(EquipmentBus) -> Merge1/4
  Switch Case2/1 -> VehicleEquipment4/Action
  In Bus Element/1 -> Data Type Conversion/1
  Switch Case2/3 -> VehicleEquipment2/Action
  Data Type Conversion/1 -> Switch Case2/1  "VehicleClasEnum"
  Switch Case2/4 -> VehicleEquipment3/Action
  Merge1/1 -> Doors/1
  Switch Case2/2 -> VehicleEquipment1/Action
  VehicleEquipment4/1(EquipmentBus) -> Merge1/1

== system BEML_EMU/InputsInterface/VehicleConfigProcessing/VehicleConfigInterface/VehicleConfigInterface/AssignElectrical ==
  In Bus Element : Inport  PortName=VehicleConfig  Element=Common.Class
  Index : Inport  Port=2
  Data Type Conversion : DataTypeConversion
  Merge1 : Merge  Inputs=4
  Switch Case2 : SwitchCase  CaseConditions={[101], [102], [103]}
  VehicleEquipment : Subsystem  mask(Tram Vehicle Equipment){HasCab=on, HasMotors=on, HasPantograph=off, HasPantoReservoir=off, HasMainCompressor=on}
      mask prompts: HasCab "Has Cab?"; HasMotors "Has Motors?"; HasPantograph "Has Pantograph?"; HasPantoReservoir "HasPantoReservoir?"
      mask DialogControl ParameterGroupVar Prompt: Equipment
  VehicleEquipment1 : Subsystem  mask(Tram Vehicle Equipment){HasCab=off, HasMotors=off, HasPantograph=on, HasPantoReservoir=on, HasMainCompressor=off}
      mask prompts: HasCab "Has Cab?"; HasMotors "Has Motors?"; HasPantograph "Has Pantograph?"; HasPantoReservoir "HasPantoReservoir?"
      mask DialogControl ParameterGroupVar Prompt: Equipment
  VehicleEquipment2 : Subsystem  mask(Tram Vehicle Equipment){HasCab=off, HasMotors=off, HasPantograph=off, HasPantoReservoir=off, HasMainCompressor=off}
      mask prompts: HasCab "Has Cab?"; HasMotors "Has Motors?"; HasPantograph "Has Pantograph?"; HasPantoReservoir "HasPantoReservoir?"
      mask DialogControl ParameterGroupVar Prompt: Equipment
  VehicleEquipment3 : Subsystem  mask(Tram Vehicle Equipment){HasCab=off, HasMotors=on, HasPantograph=off, HasPantoReservoir=off, HasMainCompressor=off}
      mask prompts: HasCab "Has Cab?"; HasMotors "Has Motors?"; HasPantograph "Has Pantograph?"; HasPantoReservoir "HasPantoReservoir?"
      mask DialogControl ParameterGroupVar Prompt: Equipment
  ElectricalBus : Outport  VectorParamsAs1DForOutWhenUnconnected=off
  wires:
  VehicleEquipment3/1(EquipmentBus) -> Merge1/3
  VehicleEquipment1/1(EquipmentBus) -> Merge1/2
  VehicleEquipment2/1(EquipmentBus) -> Merge1/4
  Switch Case2/1 -> VehicleEquipment/Action
  In Bus Element/1 -> Data Type Conversion/1
  Switch Case2/3 -> VehicleEquipment3/Action
  Data Type Conversion/1 -> Switch Case2/1  "VehicleClasEnum"
  Switch Case2/4 -> VehicleEquipment2/Action
  Merge1/1 -> ElectricalBus/1
  Switch Case2/2 -> VehicleEquipment1/Action
  VehicleEquipment/1(EquipmentBus) -> Merge1/1
  Index/1 -> VehicleEquipment3/1(Index), VehicleEquipment1/1(Index), VehicleEquipment/1(Index)

== system BEML_EMU/InputsInterface/VehicleConfigProcessing/VehicleConfigInterface/VehicleConfigInterface/AssignEquipment ==
  In Bus Element : Inport  PortName=VehicleConfig  Element=Common.Class
  Data Type Conversion : DataTypeConversion
  Merge1 : Merge  Inputs=4
  Switch Case2 : SwitchCase  CaseConditions={[101], [102], [103]}
  VehicleEquipment : Subsystem  mask(Tram Vehicle Equipment){HasCab=on, HasBogie=on, HasMotors=on, HasMainCompressor=on, HasMainReservoir=on, HasPantoReservoir=off, HasBrakeSystem=on, HasPneumaticPanto=off, HasElectricPanto=off, NumberOfDoors=8, NumberOfTractionBogies=2, NumberOfBrakingBogies=2}
      mask prompts: HasCab "Has Cab?"; HasBogie "Has Bogie?"; HasMotors "Has Motors?"; HasMainCompressor "Has Main Compressor?"; HasMainReservoir "Has Main Reservoir?"; HasPantoReservoir "Has Panto Reservoir?"; HasBrakeSystem "Has Brake System?"; HasPneumaticPanto "Has Pneumatic Panto?"; HasElectricPanto "Has Electric Panto?"; NumberOfDoors "Number Of Doors"; NumberOfTractionBogies "Number Of Traction Bogies"; NumberOfBrakingBogies "Number Of Braking Bogies"
      mask DialogControl ParameterGroupVar Prompt: Equipment
  VehicleEquipment1 : Subsystem  mask(Tram Vehicle Equipment){HasCab=off, HasBogie=on, HasMotors=off, HasMainCompressor=off, HasMainReservoir=off, HasPantoReservoir=on, HasBrakeSystem=on, HasPneumaticPanto=on, HasElectricPanto=off, NumberOfDoors=8, NumberOfTractionBogies=0, NumberOfBrakingBogies=2}
      mask prompts: HasCab "Has Cab?"; HasBogie "Has Bogie?"; HasMotors "Has Motors?"; HasMainCompressor "Has Main Compressor?"; HasMainReservoir "Has Main Reservoir?"; HasPantoReservoir "Has Panto Reservoir?"; HasBrakeSystem "Has Brake System?"; HasPneumaticPanto "Has Pneumatic Panto?"; HasElectricPanto "Has Electric Panto?"; NumberOfDoors "Number Of Doors"; NumberOfTractionBogies "Number Of Traction Bogies"; NumberOfBrakingBogies "Number Of Braking Bogies"
      mask DialogControl ParameterGroupVar Prompt: Equipment
  VehicleEquipment2 : Subsystem  mask(Tram Vehicle Equipment){HasCab=off, HasBogie=on, HasMotors=on, HasMainCompressor=off, HasMainReservoir=off, HasPantoReservoir=off, HasBrakeSystem=on, HasPneumaticPanto=off, HasElectricPanto=off, NumberOfDoors=8, NumberOfTractionBogies=2, NumberOfBrakingBogies=2}
      mask prompts: HasCab "Has Cab?"; HasBogie "Has Bogie?"; HasMotors "Has Motors?"; HasMainCompressor "Has Main Compressor?"; HasMainReservoir "Has Main Reservoir?"; HasPantoReservoir "Has Panto Reservoir?"; HasBrakeSystem "Has Brake System?"; HasPneumaticPanto "Has Pneumatic Panto?"; HasElectricPanto "Has Electric Panto?"; NumberOfDoors "Number Of Doors"; NumberOfTractionBogies "Number Of Traction Bogies"; NumberOfBrakingBogies "Number Of Braking Bogies"
      mask DialogControl ParameterGroupVar Prompt: Equipment
  VehicleEquipment3 : Subsystem  mask(Tram Vehicle Equipment){HasCab=off, HasBogie=off, HasMotors=off, HasMainCompressor=off, HasMainReservoir=off, HasPantoReservoir=off, HasBrakeSystem=off, HasPneumaticPanto=off, HasElectricPanto=off, NumberOfDoors=0, NumberOfTractionBogies=2, NumberOfBrakingBogies=2}
      mask prompts: HasCab "Has Cab?"; HasBogie "Has Bogie?"; HasMotors "Has Motors?"; HasMainCompressor "Has Main Compressor?"; HasMainReservoir "Has Main Reservoir?"; HasPantoReservoir "Has Panto Reservoir?"; HasBrakeSystem "Has Brake System?"; HasPneumaticPanto "Has Pneumatic Panto?"; HasElectricPanto "Has Electric Panto?"; NumberOfDoors "Number Of Doors"; NumberOfTractionBogies "Number Of Traction Bogies"; NumberOfBrakingBogies "Number Of Braking Bogies"
      mask DialogControl ParameterGroupVar Prompt: Equipment
  EquipmentBus : Outport  VectorParamsAs1DForOutWhenUnconnected=off
  wires:
  VehicleEquipment/1(EquipmentBus) -> Merge1/1
  Switch Case2/2 -> VehicleEquipment1/Action
  Merge1/1 -> EquipmentBus/1
  Switch Case2/4 -> VehicleEquipment3/Action
  Data Type Conversion/1 -> Switch Case2/1  "VehicleClasEnum"
  Switch Case2/3 -> VehicleEquipment2/Action
  In Bus Element/1 -> Data Type Conversion/1
  Switch Case2/1 -> VehicleEquipment/Action
  VehicleEquipment3/1(EquipmentBus) -> Merge1/4
  VehicleEquipment1/1(EquipmentBus) -> Merge1/2
  VehicleEquipment2/1(EquipmentBus) -> Merge1/3

== system BEML_EMU/InputsInterface/VehicleConfigProcessing/VehicleConfigInterface/VehicleConfigInterface/AssignPanto ==
  In Bus Element : Inport  PortName=VehicleConfig  Element=Common.Class
  Data Type Conversion : DataTypeConversion
  Merge1 : Merge  Inputs=4
  Switch Case2 : SwitchCase  CaseConditions={[101], [102], [103]}
  VehicleEquipment : Subsystem  mask(Tram Vehicle Equipment){HasPanto=off, PenumaticsPoweredPanto=off, ElectricPoweredPanto=off}
      mask prompts: HasPanto "Has Panto?"; PenumaticsPoweredPanto "Penumatics Powered Panto?"; ElectricPoweredPanto "Electric Powered Panto?"
      mask DialogControl ParameterGroupVar Prompt: Equipment
  VehicleEquipment1 : Subsystem  mask(Tram Vehicle Equipment){HasPanto=on, PenumaticsPoweredPanto=on, ElectricPoweredPanto=off}
      mask prompts: HasPanto "Has Panto?"; PenumaticsPoweredPanto "Penumatics Powered Panto?"; ElectricPoweredPanto "Electric Powered Panto?"
      mask DialogControl ParameterGroupVar Prompt: Equipment
  VehicleEquipment2 : Subsystem  mask(Tram Vehicle Equipment){HasPanto=off, PenumaticsPoweredPanto=off, ElectricPoweredPanto=off}
      mask prompts: HasPanto "Has Panto?"; PenumaticsPoweredPanto "Penumatics Powered Panto?"; ElectricPoweredPanto "Electric Powered Panto?"
      mask DialogControl ParameterGroupVar Prompt: Equipment
  VehicleEquipment3 : Subsystem  mask(Tram Vehicle Equipment){HasPanto=off, PenumaticsPoweredPanto=off, ElectricPoweredPanto=off}
      mask prompts: HasPanto "Has Panto?"; PenumaticsPoweredPanto "Penumatics Powered Panto?"; ElectricPoweredPanto "Electric Powered Panto?"
      mask DialogControl ParameterGroupVar Prompt: Equipment
  PantoBus : Outport  VectorParamsAs1DForOutWhenUnconnected=off
  wires:
  VehicleEquipment3/1(EquipmentBus) -> Merge1/3
  VehicleEquipment1/1(EquipmentBus) -> Merge1/2
  VehicleEquipment2/1(EquipmentBus) -> Merge1/4
  Switch Case2/1 -> VehicleEquipment/Action
  In Bus Element/1 -> Data Type Conversion/1
  Switch Case2/3 -> VehicleEquipment3/Action
  Data Type Conversion/1 -> Switch Case2/1  "VehicleClasEnum"
  Switch Case2/4 -> VehicleEquipment2/Action
  Merge1/1 -> PantoBus/1
  Switch Case2/2 -> VehicleEquipment1/Action
  VehicleEquipment/1(EquipmentBus) -> Merge1/1

== system BEML_EMU/InputsInterface/VehicleConfigProcessing/VehicleConfigInterface/VehicleConfigInterface/AssignPneumatics ==
  In Bus Element : Inport  PortName=VehicleConfig  Element=Common.Class
  Data Type Conversion : DataTypeConversion
  Merge1 : Merge  Inputs=4
  Switch Case2 : SwitchCase  CaseConditions={[101], [102], [103]}
  VehicleEquipment : Subsystem  mask(Tram Vehicle Equipment){HasCab=on, HasBogie=on, HasPantograph=off, HasCompressor=on, HasMainReservoir=on, HasBrakeSystem=on}
      mask prompts: HasCab "Has Cab?"; HasBogie "Has Bogie?"; HasPantograph "Has Pantograph?"; HasCompressor "Has Compressor?"; HasMainReservoir "Has Main Reservoir?"; HasBrakeSystem "Has Brake System?"
      mask DialogControl ParameterGroupVar Prompt: Equipment
  VehicleEquipment1 : Subsystem  mask(Tram Vehicle Equipment){HasCab=off, HasBogie=on, HasPantograph=on, HasCompressor=on, HasMainReservoir=off, HasBrakeSystem=on}
      mask prompts: HasCab "Has Cab?"; HasBogie "Has Bogie?"; HasPantograph "Has Pantograph?"; HasCompressor "Has Compressor?"; HasMainReservoir "Has Main Reservoir?"; HasBrakeSystem "Has Brake System?"
      mask DialogControl ParameterGroupVar Prompt: Equipment
  VehicleEquipment2 : Subsystem  mask(Tram Vehicle Equipment){HasCab=off, HasBogie=on, HasPantograph=off, HasCompressor=off, HasMainReservoir=off, HasBrakeSystem=on}
      mask prompts: HasCab "Has Cab?"; HasBogie "Has Bogie?"; HasPantograph "Has Pantograph?"; HasCompressor "Has Compressor?"; HasMainReservoir "Has Main Reservoir?"; HasBrakeSystem "Has Brake System?"
      mask DialogControl ParameterGroupVar Prompt: Equipment
  VehicleEquipment3 : Subsystem  mask(Tram Vehicle Equipment){HasCab=off, HasBogie=off, HasPantograph=off, HasCompressor=off, HasMainReservoir=off, HasBrakeSystem=off}
      mask prompts: HasCab "Has Cab?"; HasBogie "Has Bogie?"; HasPantograph "Has Pantograph?"; HasCompressor "Has Compressor?"; HasMainReservoir "Has Main Reservoir?"; HasBrakeSystem "Has Brake System?"
      mask DialogControl ParameterGroupVar Prompt: Equipment
  PneumaticsBus : Outport  VectorParamsAs1DForOutWhenUnconnected=off
  wires:
  VehicleEquipment2/1(EquipmentBus) -> Merge1/3
  VehicleEquipment1/1(EquipmentBus) -> Merge1/2
  VehicleEquipment3/1(EquipmentBus) -> Merge1/4
  Switch Case2/1 -> VehicleEquipment/Action
  In Bus Element/1 -> Data Type Conversion/1
  Switch Case2/3 -> VehicleEquipment2/Action
  Data Type Conversion/1 -> Switch Case2/1  "VehicleClasEnum"
  Switch Case2/4 -> VehicleEquipment3/Action
  Merge1/1 -> PneumaticsBus/1
  Switch Case2/2 -> VehicleEquipment1/Action
  VehicleEquipment/1(EquipmentBus) -> Merge1/1
